simulink model "RO_Plantsimscape"  (R2020a)
settings: Solver=VariableStepAuto  StartTime=0.0  StopTime=100  RelTol=1e-3
libraries: sh_lib x108, fl_lib x76, nesl_utility x73, simulink x13
(part 1 of 4)
settings Model: Creator=cjrmx  LastModifiedBy=Kevin

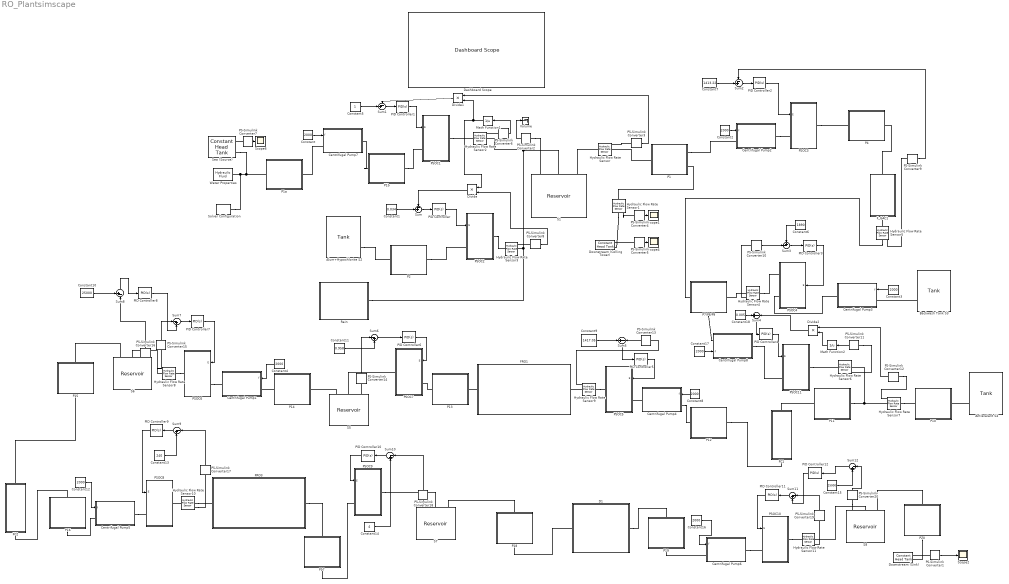
== system RO_Plantsimscape ==
  Alum+Hypochlorite S2 : sh_lib/Low-Pressure Blocks/Tank  press=1 atm  level_spec=1  tank_area=342.26 m^2  fluid_volume_tab=[0, .0028, .0065, .0114, .0176, .0252, .0344, .0436, .0512, .0574, .0623, .066, .0688, .0707, .072, .0727] m^3  fluid_level_tab=[0, .02, .04, .06, .08, .1, .12, .14, .16, .18, .2, .22, .24, .26, .28, .3] m  interp_method=1  extrap_method=1  pipe_diam=10 in  loss_coeff=1.2  g=9.81 m/s^2  min_level=1e-3 m  fluid_level_check=1  volume_specify=off  volume_priority=High  volume=20 l  volume_nominal_specify=off  volume_nominal_unit=l  volume_nominal_value=1  level_specify=on  level_priority=None  level=15 m  level_nominal_specify=off  level_nominal_unit=m  level_nominal_value=1  pipe_diam_A=0.02 m  loss_coeff_A=1.2  height_B=0.8 m  pipe_diam_B=0.02 m  loss_coeff_B=1.2  height_C=0.8 m  pipe_diam_C=0.02 m  loss_coeff_C=1.2
      settings: SourceProductBaseCode=SH  InternalSimscapePortConfiguration="{\"Bottom\":[],\"Left\":[],\"Right\":[{\"id\":\"V\",\"label\":\"V\",\"type\":\"output\"},{\"id\":\"T\",\"label\":\"T\",\"type\":\"foundation.hydraulic.hydraulic\"}],\"Top\":[]}"
  Antiscalant S4 : sh_lib/Low-Pressure Blocks/Tank  press=1 atm  level_spec=1  tank_area=20 m^2  fluid_volume_tab=[0, .0028, .0065, .0114, .0176, .0252, .0344, .0436, .0512, .0574, .0623, .066, .0688, .0707, .072, .0727] m^3  fluid_level_tab=[0, .02, .04, .06, .08, .1, .12, .14, .16, .18, .2, .22, .24, .26, .28, .3] m  interp_method=1  extrap_method=1  pipe_diam=0.02 m  loss_coeff=1.2  g=9.81 m/s^2  min_level=1e-3 m  fluid_level_check=1  volume_specify=off  volume_priority=High  volume=20 l  volume_nominal_specify=off  volume_nominal_unit=l  volume_nominal_value=1  level_specify=on  level_priority=None  level=12 m  level_nominal_specify=off  level_nominal_unit=m  level_nominal_value=1  pipe_diam_A=0.02 m  loss_coeff_A=1.2  height_B=0.8 m  pipe_diam_B=0.02 m  loss_coeff_B=1.2  height_C=0.8 m  pipe_diam_C=0.02 m  loss_coeff_C=1.2
      settings: SourceProductBaseCode=SH  InternalSimscapePortConfiguration="{\"Bottom\":[],\"Left\":[],\"Right\":[{\"id\":\"V\",\"label\":\"V\",\"type\":\"output\"},{\"id\":\"T\",\"label\":\"T\",\"type\":\"foundation.hydraulic.hydraulic\"}],\"Top\":[]}"
  Backwash Tank S3 : sh_lib/Low-Pressure Blocks/Tank  press=1 atm  level_spec=1  tank_area=12.57 m^2  fluid_volume_tab=[0, .0028, .0065, .0114, .0176, .0252, .0344, .0436, .0512, .0574, .0623, .066, .0688, .0707, .072, .0727] m^3  fluid_level_tab=[0, .02, .04, .06, .08, .1, .12, .14, .16, .18, .2, .22, .24, .26, .28, .3] m  interp_method=1  extrap_method=1  pipe_diam=0.02 m  loss_coeff=1.2  g=9.81 m/s^2  min_level=1e-3 m  fluid_level_check=1  volume_specify=off  volume_priority=High  volume=20 l  volume_nominal_specify=off  volume_nominal_unit=l  volume_nominal_value=1  level_specify=on  level_priority=None  level=8 m  level_nominal_specify=off  level_nominal_unit=m  level_nominal_value=1  pipe_diam_A=0.02 m  loss_coeff_A=1.2  height_B=0.8 m  pipe_diam_B=0.02 m  loss_coeff_B=1.2  height_C=0.8 m  pipe_diam_C=0.02 m  loss_coeff_C=1.2
      settings: SourceProductBaseCode=SH  InternalSimscapePortConfiguration="{\"Bottom\":[],\"Left\":[],\"Right\":[{\"id\":\"V\",\"label\":\"V\",\"type\":\"output\"},{\"id\":\"T\",\"label\":\"T\",\"type\":\"foundation.hydraulic.hydraulic\"}],\"Top\":[]}"
  Centrifugal Pump1 : Subsystem
      mask Display: image('$imagefile'); % Use "Edit Image" on toolstrip to change.
  Centrifugal Pump2 : Subsystem
      mask Display: image('$imagefile'); % Use "Edit Image" on toolstrip to change.
  Centrifugal Pump3 : Subsystem
      mask Display: image('$imagefile'); % Use "Edit Image" on toolstrip to change.
  Centrifugal Pump4 : Subsystem
      mask Display: image('$imagefile'); % Use "Edit Image" on toolstrip to change.
  Centrifugal Pump5 : Subsystem
      mask Display: image('$imagefile'); % Use "Edit Image" on toolstrip to change.
  Centrifugal Pump6 : Subsystem
      mask Display: image('$imagefile'); % Use "Edit Image" on toolstrip to change.
  Centrifugal Pump7 : Subsystem
      mask Display: image('$imagefile'); % Use "Edit Image" on toolstrip to change.
  Centrifugal Pump8 : Subsystem
      settings: PortSchema="{\"entries\":[{\"content\":{\"sides\":[{\"content\":{\"connectorIds\":[\"LConn1\",\"In1\"]},\"type\":\"ConnectorPlacement.EquallySpacedRectSide\",\"uuid\":\"eab26e76-19e5-4131-be01-7f1e86a3578c\"},{\"content\":{\"connectorIds\":[\"RConn1\"],\"side\":\"RIGHT\"},\"type\":\"ConnectorPlacement.EquallySpacedRectSide\",\"uuid\":\"eb3e9ef5-afdc-4988-b145-41f6f9d64aea\"},{\"content\":{\"connectorIds\":[],\"side\":\"TOP\"},\"type\":\"ConnectorPlacement.EquallySpacedRectSide\",\"uuid\":\"3eed5e1d-ef70-4ff8-841b-e6ca0040c613\"}]},\"type\":\"ConnectorPlacement.EquallySpacedConnector\",\"uuid\":\"4f5dbfc8-7a84-4fdf-87d5-9a92094a984d\"}],\"packageUris\":[\"http://schema.mathworks.com/mf0/Connector/19700101\"],\"version\":\"1.0\"}"
      mask Display: image('$imagefile'); % Use "Edit Image" on toolstrip to change.
  Constant{,2..4,8,12,16..17} (8 alike) : Constant  Value=2000
  Constant1 : Constant  Value=0.034
  Constant10 : Constant  Value=25000
  Constant11 : Constant  Value=0.958
  Constant13 : Constant  Value=240
  Constant14 : Constant  Value=4
  Constant15 : Constant  Value=25000
  Constant18 : Constant  Value=0.005
  Constant5 : Constant
  Constant6 : Constant  Value=1890
  Constant7 : Constant  Value=1413.22
  Constant9 : Constant  Value=1417.05
  D1 : Subsystem
      mask Display: image('$imagefile'); % Use "Edit Image" on toolstrip to change.
  Dashboard Scope : DashboardScope
  Divide : Product  Inputs=**
  Divide1 : Product  Inputs=**
  Divide2 : Product  Inputs=**
  Downstream (Colling Tower) : sh_lib/Low-Pressure Blocks/Constant Head Tank  press=0 Pa  fluid_level=0 m  pipe_diam=48 in  loss_coeff=1.2  g=9.81 m/s^2  volume_specify=on  volume_priority=High  volume=0 m^3  volume_nominal_specify=off  volume_nominal_unit=m^3  volume_nominal_value=1
      settings: SourceProductBaseCode=SH  InternalSimscapePortConfiguration="{\"Bottom\":[],\"Left\":[],\"Right\":[{\"id\":\"V\",\"label\":\"V\",\"type\":\"output\"},{\"id\":\"T\",\"label\":\"T\",\"type\":\"foundation.hydraulic.hydraulic\"}],\"Top\":[]}"
  Downstream (Sink) : sh_lib/Low-Pressure Blocks/Constant Head Tank  press=0 Pa  fluid_level=0 m  pipe_diam=4 in  loss_coeff=1.2  g=9.81 m/s^2  volume_specify=on  volume_priority=High  volume=0 m^3  volume_nominal_specify=off  volume_nominal_unit=m^3  volume_nominal_value=1
      settings: SourceProductBaseCode=SH  InternalSimscapePortConfiguration="{\"Bottom\":[],\"Left\":[],\"Right\":[{\"id\":\"V\",\"label\":\"V\",\"type\":\"output\"},{\"id\":\"T\",\"label\":\"T\",\"type\":\"foundation.hydraulic.hydraulic\"}],\"Top\":[]}"
  FC1 : Subsystem
      mask Display: image('$imagefile'); % Use "Edit Image" on toolstrip to change.
  FC2 : Subsystem
      mask Display: image('$imagefile'); % Use "Edit Image" on toolstrip to change.
  FRO1 : Subsystem
      mask Display: image('$imagefile'); % Use "Edit Image" on toolstrip to change.
  FRO3 : Subsystem
      mask Display: image('$imagefile'); % Use "Edit Image" on toolstrip to change.
  F_GAC1 : Subsystem
      mask Display: image('$imagefile'); % Use "Edit Image" on toolstrip to change.
  Hydraulic Flow Rate Sensor{,1..11} (12 alike) : fl_lib/Hydraulic/Hydraulic Sensors/Hydraulic Flow Rate Sensor
  Math Function1 : Math  Operator=reciprocal  SaturateOnIntegerOverflow=on
  Math Function2 : Math  Operator=reciprocal  SaturateOnIntegerOverflow=on
  P1 : Subsystem
      mask Display: image('$imagefile'); % Use "Edit Image" on toolstrip to change.
  P10 : Subsystem
      mask Display: image('$imagefile'); % Use "Edit Image" on toolstrip to change.
  P11 : Subsystem
      mask Display: image('$imagefile'); % Use "Edit Image" on toolstrip to change.
  P12 : Subsystem
      mask Display: image('$imagefile'); % Use "Edit Image" on toolstrip to change.
  P13 : Subsystem
      mask Display: image('$imagefile'); % Use "Edit Image" on toolstrip to change.
  P14 : Subsystem
      mask Display: image('$imagefile'); % Use "Edit Image" on toolstrip to change.
  P15 : Subsystem
      settings: PortSchema="{\"entries\":[{\"content\":{\"sides\":[{\"content\":{\"connectorIds\":[]},\"type\":\"ConnectorPlacement.EquallySpacedRectSide\",\"uuid\":\"46c43a71-b7fa-42e4-8d4f-3c01e3706290\"},{\"content\":{\"connectorIds\":[],\"side\":\"RIGHT\"},\"type\":\"ConnectorPlacement.EquallySpacedRectSide\",\"uuid\":\"b401084b-7303-4528-8d6f-c80864bdaeba\"},{\"content\":{\"connectorIds\":[\"LConn1\"],\"side\":\"TOP\"},\"type\":\"ConnectorPlacement.EquallySpacedRectSide\",\"uuid\":\"e7f94297-9de0-49cb-bb6c-7569d7bc8c1f\"},{\"content\":{\"connectorIds\":[\"RConn1\"],\"side\":\"BOTTOM\"},\"type\":\"ConnectorPlacement.EquallySpacedRectSide\",\"uuid\":\"17d2f97d-9159-4642-b3f0-323a39ef2445\"}]},\"type\":\"ConnectorPlacement.EquallySpacedConnector\",\"uuid\":\"a507a281-e5f3-478b-81a6-535710a561dc\"}],\"packageUris\":[\"http://schema.mathworks.com/mf0/Connector/19700101\"],\"version\":\"1.0\"}"
      mask Display: image('$imagefile'); % Use "Edit Image" on toolstrip to change.
  P16 : Subsystem
      settings: PortSchema="{\"entries\":[{\"content\":{\"sides\":[{\"content\":{\"connectorIds\":[]},\"type\":\"ConnectorPlacement.EquallySpacedRectSide\",\"uuid\":\"46c43a71-b7fa-42e4-8d4f-3c01e3706290\"},{\"content\":{\"connectorIds\":[],\"side\":\"RIGHT\"},\"type\":\"ConnectorPlacement.EquallySpacedRectSide\",\"uuid\":\"b401084b-7303-4528-8d6f-c80864bdaeba\"},{\"content\":{\"connectorIds\":[\"LConn1\"],\"side\":\"TOP\"},\"type\":\"ConnectorPlacement.EquallySpacedRectSide\",\"uuid\":\"e7f94297-9de0-49cb-bb6c-7569d7bc8c1f\"},{\"content\":{\"connectorIds\":[\"RConn1\"],\"side\":\"BOTTOM\"},\"type\":\"ConnectorPlacement.EquallySpacedRectSide\",\"uuid\":\"17d2f97d-9159-4642-b3f0-323a39ef2445\"}]},\"type\":\"ConnectorPlacement.EquallySpacedConnector\",\"uuid\":\"a507a281-e5f3-478b-81a6-535710a561dc\"}],\"packageUris\":[\"http://schema.mathworks.com/mf0/Connector/19700101\"],\"version\":\"1.0\"}"
      mask Display: image('$imagefile'); % Use "Edit Image" on toolstrip to change.
  P17 : Subsystem
      settings: PortSchema="{\"entries\":[{\"content\":{\"sides\":[{\"content\":{\"connectorIds\":[]},\"type\":\"ConnectorPlacement.EquallySpacedRectSide\",\"uuid\":\"46c43a71-b7fa-42e4-8d4f-3c01e3706290\"},{\"content\":{\"connectorIds\":[],\"side\":\"RIGHT\"},\"type\":\"ConnectorPlacement.EquallySpacedRectSide\",\"uuid\":\"b401084b-7303-4528-8d6f-c80864bdaeba\"},{\"content\":{\"connectorIds\":[\"LConn1\"],\"side\":\"TOP\"},\"type\":\"ConnectorPlacement.EquallySpacedRectSide\",\"uuid\":\"e7f94297-9de0-49cb-bb6c-7569d7bc8c1f\"},{\"content\":{\"connectorIds\":[\"RConn1\"],\"side\":\"BOTTOM\"},\"type\":\"ConnectorPlacement.EquallySpacedRectSide\",\"uuid\":\"17d2f97d-9159-4642-b3f0-323a39ef2445\"}]},\"type\":\"ConnectorPlacement.EquallySpacedConnector\",\"uuid\":\"a507a281-e5f3-478b-81a6-535710a561dc\"}],\"packageUris\":[\"http://schema.mathworks.com/mf0/Connector/19700101\"],\"version\":\"1.0\"}"
      mask Display: image('$imagefile'); % Use "Edit Image" on toolstrip to change.
  P18 : Subsystem
      settings: PortSchema="{\"entries\":[{\"content\":{\"sides\":[{\"content\":{\"connectorIds\":[]},\"type\":\"ConnectorPlacement.EquallySpacedRectSide\",\"uuid\":\"46c43a71-b7fa-42e4-8d4f-3c01e3706290\"},{\"content\":{\"connectorIds\":[],\"side\":\"RIGHT\"},\"type\":\"ConnectorPlacement.EquallySpacedRectSide\",\"uuid\":\"b401084b-7303-4528-8d6f-c80864bdaeba\"},{\"content\":{\"connectorIds\":[\"LConn1\"],\"side\":\"TOP\"},\"type\":\"ConnectorPlacement.EquallySpacedRectSide\",\"uuid\":\"e7f94297-9de0-49cb-bb6c-7569d7bc8c1f\"},{\"content\":{\"connectorIds\":[\"RConn1\"],\"side\":\"BOTTOM\"},\"type\":\"ConnectorPlacement.EquallySpacedRectSide\",\"uuid\":\"17d2f97d-9159-4642-b3f0-323a39ef2445\"}]},\"type\":\"ConnectorPlacement.EquallySpacedConnector\",\"uuid\":\"a507a281-e5f3-478b-81a6-535710a561dc\"}],\"packageUris\":[\"http://schema.mathworks.com/mf0/Connector/19700101\"],\"version\":\"1.0\"}"
      mask Display: image('$imagefile'); % Use "Edit Image" on toolstrip to change.
  P19 : Subsystem
      settings: PortSchema="{\"entries\":[{\"content\":{\"sides\":[{\"content\":{\"connectorIds\":[]},\"type\":\"ConnectorPlacement.EquallySpacedRectSide\",\"uuid\":\"46c43a71-b7fa-42e4-8d4f-3c01e3706290\"},{\"content\":{\"connectorIds\":[],\"side\":\"RIGHT\"},\"type\":\"ConnectorPlacement.EquallySpacedRectSide\",\"uuid\":\"b401084b-7303-4528-8d6f-c80864bdaeba\"},{\"content\":{\"connectorIds\":[\"LConn1\"],\"side\":\"TOP\"},\"type\":\"ConnectorPlacement.EquallySpacedRectSide\",\"uuid\":\"e7f94297-9de0-49cb-bb6c-7569d7bc8c1f\"},{\"content\":{\"connectorIds\":[\"RConn1\"],\"side\":\"BOTTOM\"},\"type\":\"ConnectorPlacement.EquallySpacedRectSide\",\"uuid\":\"17d2f97d-9159-4642-b3f0-323a39ef2445\"}]},\"type\":\"ConnectorPlacement.EquallySpacedConnector\",\"uuid\":\"a507a281-e5f3-478b-81a6-535710a561dc\"}],\"packageUris\":[\"http://schema.mathworks.com/mf0/Connector/19700101\"],\"version\":\"1.0\"}"
      mask Display: image('$imagefile'); % Use "Edit Image" on toolstrip to change.
  P1a : Subsystem
      mask Display: image('$imagefile'); % Use "Edit Image" on toolstrip to change.
  P1b : Subsystem
      mask Display: image('$imagefile'); % Use "Edit Image" on toolstrip to change.
  P2 : Subsystem
      mask Display: image('$imagefile'); % Use "Edit Image" on toolstrip to change.
  P20 : Subsystem
      settings: PortSchema="{\"entries\":[{\"content\":{\"sides\":[{\"content\":{\"connectorIds\":[]},\"type\":\"ConnectorPlacement.EquallySpacedRectSide\",\"uuid\":\"46c43a71-b7fa-42e4-8d4f-3c01e3706290\"},{\"content\":{\"connectorIds\":[],\"side\":\"RIGHT\"},\"type\":\"ConnectorPlacement.EquallySpacedRectSide\",\"uuid\":\"b401084b-7303-4528-8d6f-c80864bdaeba\"},{\"content\":{\"connectorIds\":[\"LConn1\"],\"side\":\"TOP\"},\"type\":\"ConnectorPlacement.EquallySpacedRectSide\",\"uuid\":\"e7f94297-9de0-49cb-bb6c-7569d7bc8c1f\"},{\"content\":{\"connectorIds\":[\"RConn1\"],\"side\":\"BOTTOM\"},\"type\":\"ConnectorPlacement.EquallySpacedRectSide\",\"uuid\":\"17d2f97d-9159-4642-b3f0-323a39ef2445\"}]},\"type\":\"ConnectorPlacement.EquallySpacedConnector\",\"uuid\":\"a507a281-e5f3-478b-81a6-535710a561dc\"}],\"packageUris\":[\"http://schema.mathworks.com/mf0/Connector/19700101\"],\"version\":\"1.0\"}"
      mask Display: image('$imagefile'); % Use "Edit Image" on toolstrip to change.
  P4 : Subsystem
      mask Display: image('$imagefile'); % Use "Edit Image" on toolstrip to change.
  P7/P8/P9 : Subsystem
      settings: PortSchema="{\"entries\":[{\"content\":{\"sides\":[{\"content\":{\"connectorIds\":[\"LConn1\"]},\"type\":\"ConnectorPlacement.EquallySpacedRectSide\",\"uuid\":\"c4d3b345-1774-4faf-92d9-0d4f63b9ee50\"},{\"content\":{\"connectorIds\":[\"RConn1\"],\"side\":\"RIGHT\"},\"type\":\"ConnectorPlacement.EquallySpacedRectSide\",\"uuid\":\"19590d96-e8de-4e96-ac4d-d2cb11dc0057\"},{\"content\":{\"connectorIds\":[],\"side\":\"TOP\"},\"type\":\"ConnectorPlacement.EquallySpacedRectSide\",\"uuid\":\"ab799575-47ef-4b74-8840-5dcb81dec600\"},{\"content\":{\"connectorIds\":[\"RConn2\"],\"side\":\"BOTTOM\"},\"type\":\"ConnectorPlacement.EquallySpacedRectSide\",\"uuid\":\"f791b078-7d26-4714-95a8-19c732dd4143\"}]},\"type\":\"ConnectorPlacement.EquallySpacedConnector\",\"uuid\":\"41b3ff9f-9b96-49e2-b98d-ecd42f4aada1\"}],\"packageUris\":[\"http://schema.mathworks.com/mf0/Connector/19700101\"],\"version\":\"1.0\"}"
      mask Display: image('$imagefile'); % Use "Edit Image" on toolstrip to change.
  PID Controller{,1..12} (13 alike) : simulink/Continuous/PID Controller  Controller=PID  Form=Parallel  TimeDomain=Continuous-time  UseExternalTs=off  SampleTime=-1  IntegratorMethod=Forward Euler  FilterMethod=Forward Euler  ControllerParametersSource=internal  P=1  I=1  D=0  UseFilter=on  N=100  TunerSelectOption=Transfer Function Based (PID Tuner App)  InitialConditionSource=internal  InitialConditionForIntegrator=0  InitialConditionForFilter=0  DifferentiatorICPrevScaledInput=0  ExternalReset=none  TrackingMode=off  Kt=1  LimitOutput=off  UpperSaturationLimit=inf  LowerSaturationLimit=-inf  LinearizeAsGain=on  AntiWindupMode=none  Kb=1  POutMin=[]  POutMax=[]  IOutMin=[]  IOutMax=[]  DOutMin=[]  DOutMax=[]  NOutMin=[]  NOutMax=[]  SumOutMin=[]  SumOutMax=[]  SaturationOutMin=[]  SaturationOutMax=[]  PParamMin=[]  PParamMax=[]  IParamMin=[]  IParamMax=[]  DParamMin=[]  DParamMax=[]  NParamMin=[]  NParamMax=[]  KbParamMin=[]  KbParamMax=[]  KtParamMin=[]  KtParamMax=[]  KbOutMin=[]  KbOutMax=[]  KtOutMin=[]  KtOutMax=[]  IntegratorOutMin=[]  IntegratorOutMax=[]  FilterOutMin=[]  FilterOutMax=[]  SumI1OutMin=[]  SumI1OutMax=[]  SumI2OutMin=[]  SumI2OutMax=[]  SumI3OutMin=[]  SumI3OutMax=[]  SumI4OutMin=[]  SumI4OutMax=[]  SumDOutMin=[]  SumDOutMax=[]  DifferentiatorOutMin=[]  DifferentiatorOutMax=[]  FilterDiffOutCoefMin=[]  FilterDiffOutCoefMax=[]  ReciprocalOutMin=[]  ReciprocalOutMax=[]  SumDenOutMin=[]  SumDenOutMax=[]  SumNumOutMin=[]  SumNumOutMax=[]  DivideOutMin=[]  DivideOutMax=[]  UdiffTsProdOutMin=[]  UdiffTsProdOutMax=[]  NTsProdOutMin=[]  NTsProdOutMax=[]  UintegralTsProdOutMin=[]  UintegralTsProdOutMax=[]  UngainTsProdOutMin=[]  UngainTsProdOutMax=[]  IntegratorContinuousStateAttributes=''  IntegratorStateMustResolveToSignalObject=off  IntegratorRTWStateStorageClass=Auto  FilterContinuousStateAttributes=''  FilterStateMustResolveToSignalObject=off  FilterRTWStateStorageClass=Auto  ParallelPVariant=InternalParameters  IdealPVariant=Disabled  IVariant=InternalParameters  DVariant=InternalParameters  IntegratorVariant=Continuous  SatVariant=Disabled  AWVariant=Passthrough  PCopyVariant=Disabled  TRVariant=Disabled  FdbkBlocksVariant=Forward  IdealPFdbkVariant=Disabled  SatFdbkVariant=Disabled  DerivativeFilterVariant=ContFilter  NVariant=InternalParameters  NCopyVariant=Disabled  FilterICVariant=InternalICsFilter  IntegratorICVariant=InternalICs  ExternalResetVariant=Disabled  TRSumVariant=Passthrough  SumFdbkVariant=Disabled  SumVariant=Sum_PID  TsampFilterVariant=InternalTs  TsampNgainVariant=Passthrough  TsampIntegralVariant=Passthrough
  PS-Simulink Converter{1..20} (20 alike) : nesl_utility/PS-Simulink Converter  PhysicalDomain=network_engine_domain  SubClassName=ps_output  LeftPortType=input  RightPortType=output  PseudoPeriodic=off  Frequencies=[]  Unit=1  AffineConversion=off
  PSOC1 : Subsystem
      mask Display: image('$imagefile'); % Use "Edit Image" on toolstrip to change.
  PSOC10 : Subsystem
      mask Display: image('$imagefile'); % Use "Edit Image" on toolstrip to change.
  PSOC11 : Subsystem
      mask Display: image('$imagefile'); % Use "Edit Image" on toolstrip to change.
  PSOC2 : Subsystem
      mask Display: image('$imagefile'); % Use "Edit Image" on toolstrip to change.
  PSOC3 : Subsystem
      mask Display: image('$imagefile'); % Use "Edit Image" on toolstrip to change.
  PSOC4 : Subsystem
      mask Display: image('$imagefile'); % Use "Edit Image" on toolstrip to change.
  PSOC5 : Subsystem
      mask Display: image('$imagefile'); % Use "Edit Image" on toolstrip to change.
  PSOC6 : Subsystem
      mask Display: image('$imagefile'); % Use "Edit Image" on toolstrip to change.
  PSOC7 : Subsystem
      mask Display: image('$imagefile'); % Use "Edit Image" on toolstrip to change.
  PSOC8 : Subsystem
      mask Display: image('$imagefile'); % Use "Edit Image" on toolstrip to change.
  PSOC9 : Subsystem
      mask Display: image('$imagefile'); % Use "Edit Image" on toolstrip to change.
  Rain : Subsystem
      mask Display: image('$imagefile'); % Use "Edit Image" on toolstrip to change.
  S1 : sh_lib/Hydraulic Utilities/Reservoir  press=1 atm  init_volume=20000 m^3  ret_diam=48 in  loss_coeff=1
      settings: SourceProductBaseCode=SH  InternalSimscapePortConfiguration="{\"Bottom\":[],\"Left\":[{\"id\":\"V\",\"label\":\"V\",\"type\":\"output\"},{\"id\":\"P\",\"label\":\"P\",\"type\":\"foundation.hydraulic.hydraulic\"},{\"id\":\"R\",\"label\":\"R\",\"type\":\"foundation.hydraulic.hydraulic\"}],\"Right\":[],\"Top\":[]}"
  S5 : sh_lib/Hydraulic Utilities/Reservoir  press=1 atm  init_volume=1 m^3  ret_diam=4 in  loss_coeff=1
      settings: SourceProductBaseCode=SH  InternalSimscapePortConfiguration="{\"Bottom\":[],\"Left\":[{\"id\":\"V\",\"label\":\"V\",\"type\":\"output\"},{\"id\":\"P\",\"label\":\"P\",\"type\":\"foundation.hydraulic.hydraulic\"},{\"id\":\"R\",\"label\":\"R\",\"type\":\"foundation.hydraulic.hydraulic\"}],\"Right\":[],\"Top\":[]}"
  S6 : sh_lib/Hydraulic Utilities/Reservoir  press=1 atm  init_volume=27000 m^3  ret_diam=4 in  loss_coeff=1
      settings: SourceProductBaseCode=SH  InternalSimscapePortConfiguration="{\"Bottom\":[],\"Left\":[{\"id\":\"V\",\"label\":\"V\",\"type\":\"output\"},{\"id\":\"P\",\"label\":\"P\",\"type\":\"foundation.hydraulic.hydraulic\"},{\"id\":\"R\",\"label\":\"R\",\"type\":\"foundation.hydraulic.hydraulic\"}],\"Right\":[],\"Top\":[]}"
  S7 : sh_lib/Hydraulic Utilities/Reservoir  press=1 atm  init_volume=4 m^3  ret_diam=4 in  loss_coeff=1
      settings: SourceProductBaseCode=SH  InternalSimscapePortConfiguration="{\"Bottom\":[],\"Left\":[{\"id\":\"V\",\"label\":\"V\",\"type\":\"output\"},{\"id\":\"P\",\"label\":\"P\",\"type\":\"foundation.hydraulic.hydraulic\"},{\"id\":\"R\",\"label\":\"R\",\"type\":\"foundation.hydraulic.hydraulic\"}],\"Right\":[],\"Top\":[]}"
  S8 : sh_lib/Hydraulic Utilities/Reservoir  press=1 atm  init_volume=27000 m^3  ret_diam=4 in  loss_coeff=1
      settings: SourceProductBaseCode=SH  InternalSimscapePortConfiguration="{\"Bottom\":[],\"Left\":[{\"id\":\"V\",\"label\":\"V\",\"type\":\"output\"},{\"id\":\"P\",\"label\":\"P\",\"type\":\"foundation.hydraulic.hydraulic\"},{\"id\":\"R\",\"label\":\"R\",\"type\":\"foundation.hydraulic.hydraulic\"}],\"Right\":[],\"Top\":[]}"
  Scope{1..2,4,6} (4 alike) : Scope
  Sea (Source) : sh_lib/Low-Pressure Blocks/Constant Head Tank  press=1 atm  fluid_level=5000 m  pipe_diam=48 in  loss_coeff=1.2  g=9.81 m/s^2  volume_specify=on  volume_priority=High  volume=10000 m^3  volume_nominal_specify=off  volume_nominal_unit=m^3  volume_nominal_value=1
      settings: SourceProductBaseCode=SH  InternalSimscapePortConfiguration="{\"Bottom\":[],\"Left\":[],\"Right\":[{\"id\":\"V\",\"label\":\"V\",\"type\":\"output\"},{\"id\":\"T\",\"label\":\"T\",\"type\":\"foundation.hydraulic.hydraulic\"}],\"Top\":[]}"
  Solver Configuration : nesl_utility/Solver Configuration  PhysicalDomain=network_engine_domain  SubClassName=solver  LeftPortType=input  RightPortType=generic  Tones=[]  Harmonics=[]  SimulateNoise=off  Profile=off  UseLocalSampling=off  EnableSwitchedLinearOptims=on  FrequencyDomain=off  UseCCode=off  RelTol=0.001  AbsTol=1e-06  MinStep=1e-09  ToWorkspace=off  RevertToSquareIcSolve=off  NumHomotopyIterations=100  PhasorMode=off  PhasorModeNumHarmonics=1  DoDC=off  ResidualTolerance=1e-9  UseLocalSolver=off  LocalSolverChoice=NE_BACKWARD_EULER_ADVANCER  LocalSolverSampleTime=.001  DoFixedCost=off  MaxNonlinIter=3  MaxModeIter=2  LinearAlgebra=auto  EquationFormulation=NE_TIME_EF  DelaysMemoryBudget=1024  AutomaticFiltering=on  FilteringTimeConstant=0.001  PartitionStorageMethod=AS_NEEDED  PartitionMemoryBudget=1024  PartitionMethod=FAST
  Sum : Sum  Inputs=-+|
  Sum1 : Sum  Inputs=-+|
  Sum{6..7,9..12} (6 alike) : Sum  Inputs=|-+
  Sum2 : Sum  Inputs=-+|
  Sum3 : Sum  Inputs=+-|
  Sum4 : Sum  Inputs=+|-
  Sum5 : Sum  Inputs=+|-
  Sum8 : Sum  Inputs=+-|
  Volume : Terminator
  Water Properties : sh_lib/Hydraulic Utilities/Hydraulic Fluid  DataSource=1  SelFluid=24  SysTemp=1  TrapAir=0.001  ViscDerFactor=1  range_error=2
  wires:
  Constant/1 -> Centrifugal Pump7/1(f)
  PS-Simulink Converter1/1 -> Scope2/1
  PS-Simulink Converter3/1 -> Divide1/1
  PS-Simulink Converter2/1 -> Volume/1
  PS-Simulink Converter4/1 -> Scope1/1
  PS-Simulink Converter5/1 -> Scope4/1
  Constant3/1 -> Centrifugal Pump3/1(f)
  Constant8/1 -> Centrifugal Pump4/1(f)
  Constant4/1 -> Centrifugal Pump1/1(f)
  Constant12/1 -> Centrifugal Pump5/1(f)
  Constant16/1 -> Centrifugal Pump6/1(f)
  PS-Simulink Converter7/1 -> Scope6/1
  PS-Simulink Converter6/1 -> Math Function1/1
  Constant2/1 -> Centrifugal Pump2/1(f)
  Constant1/1 -> Sum/2
  Sum/1 -> PID Controller/1
  PID Controller/1 -> PSOC2/1(E)
  Divide/1 -> Sum/1
  PS-Simulink Converter8/1 -> Divide/2
  Math Function1/1 -> Divide1/2, Divide/1
  Sum1/1 -> PID Controller1/1
  Constant5/1 -> Sum1/2
  PID Controller1/1 -> PSOC1/1(E)
  Divide1/1 -> Sum1/1
  Constant7/1 -> Sum2/2
  Sum2/1 -> PID Controller2/1
  PID Controller2/1 -> PSOC3/1(E)
  PS-Simulink Converter9/1 -> Sum2/1
  PS-Simulink Converter10/1 -> Sum3/2
  Constant6/1 -> Sum3/1
  Sum3/1 -> PID Controller3/1
  PID Controller3/1 -> PSOC4/1(E)
  Constant17/1 -> Centrifugal Pump8/1(f)
  PID Controller4/1 -> PSOC11/1(E)
  Sum4/1 -> PID Controller4/1
  Constant18/1 -> Sum4/1
  PS-Simulink Converter11/1 -> Math Function2/1
  Divide2/1 -> Sum4/2
  Math Function2/1 -> Divide2/2
  PS-Simulink Converter12/1 -> Divide2/1
  PID Controller5/1 -> PSOC5/1(E)
  Sum5/1 -> PID Controller5/1
  Constant9/1 -> Sum5/1
  PS-Simulink Converter13/1 -> Sum5/2
  PID Controller6/1 -> PSOC7/1(E)
  Sum6/1 -> PID Controller6/1
  PS-Simulink Converter14/1 -> Sum6/1
  Constant11/1 -> Sum6/2
  PID Controller7/1 -> PSOC6/1(E)
  PS-Simulink Converter15/1 -> Sum7/1
  Sum7/1 -> PID Controller7/1
  PID Controller8/1 -> Sum7/2
  Sum8/1 -> PID Controller8/1
  PS-Simulink Converter16/1 -> Sum8/2
  Constant10/1 -> Sum8/1
  PS-Simulink Converter17/1 -> Sum9/1
  Sum9/1 -> PID Controller9/1
  PID Controller9/1 -> PSOC8/1(E)
  Constant13/1 -> Sum9/2
  PS-Simulink Converter18/1 -> Sum10/1
  Sum10/1 -> PID Controller10/1
  PID Controller10/1 -> PSOC9/1(E)
  Constant14/1 -> Sum10/2
  Sum11/1 -> PID Controller11/1
  PS-Simulink Converter19/1 -> Sum11/1
  PID Controller11/1 -> PSOC10/1(E)
  PS-Simulink Converter20/1 -> Sum12/1
  Sum12/1 -> PID Controller12/1
  PID Controller12/1 -> Sum11/2
  Constant15/1 -> Sum12/2
  connections:
  PS-Simulink Converter2/LConn1 -- S1/LConn1
  PS-Simulink Converter1/LConn1 -- Downstream (Sink)/RConn1
  PS-Simulink Converter3/LConn1 -- Hydraulic Flow Rate Sensor/RConn1
  Sea (Source)/RConn2 -- P1a/LConn1 -- Solver Configuration/RConn1 -- Water Properties/RConn1
  P11/LConn1 -- Hydraulic Flow Rate Sensor7/RConn2 -- Hydraulic Flow Rate Sensor6/RConn2
  Alum+Hypochlorite S2/RConn2 -- P2/LConn1
  P2/RConn1 -- PSOC2/LConn1
  Hydraulic Flow Rate Sensor1/RConn1 -- PS-Simulink Converter4/LConn1
  Hydraulic Flow Rate Sensor1/RConn2 -- Downstream (Colling Tower)/RConn2
  PS-Simulink Converter5/LConn1 -- Downstream (Colling Tower)/RConn1
  PSOC3/RConn1 -- P4/LConn1
  Centrifugal Pump3/RConn1 -- PSOC4/RConn2
  Backwash Tank S3/RConn2 -- Centrifugal Pump3/LConn1
  Antiscalant S4/RConn2 -- P10/LConn1
  P11/RConn1 -- FC1/LConn1
  P12/LConn1 -- FC1/RConn1
  S5/LConn3 -- P14/LConn1
  Centrifugal Pump4/LConn1 -- P12/RConn1
  Centrifugal Pump4/RConn1 -- PSOC5/LConn1
  PSOC6/LConn1 -- Centrifugal Pump1/RConn1
  P14/RConn1 -- Centrifugal Pump1/LConn1
  P13/RConn1 -- PSOC7/LConn1
  PSOC7/RConn1 -- S5/LConn2
  S6/LConn3 -- P15/LConn1
  FC2/LConn1 -- P15/RConn1
  Centrifugal Pump5/RConn1 -- PSOC8/LConn1
  PSOC9/RConn1 -- S7/LConn2
  Centrifugal Pump6/RConn1 -- PSOC10/LConn1
  P16/LConn1 -- FC2/RConn1
  P16/RConn1 -- Centrifugal Pump5/LConn1
  FRO3/RConn1 -- P17/LConn1
  P17/RConn1 -- PSOC9/LConn1
  S7/LConn3 -- P18/LConn1
  P18/RConn1 -- D1/LConn1
  P19/RConn1 -- Centrifugal Pump6/LConn1
  P20/RConn1 -- Downstream (Sink)/RConn2
  Hydraulic Flow Rate Sensor3/RConn2 -- Rain/RConn1 -- S1/LConn2 -- Hydraulic Flow Rate Sensor2/RConn2
  Hydraulic Flow Rate Sensor/LConn1 -- S1/LConn3
  PS-Simulink Converter7/LConn1 -- Sea (Source)/RConn1
  PSOC1/RConn1 -- Hydraulic Flow Rate Sensor2/LConn1
  Centrifugal Pump7/LConn1 -- P1a/RConn1
  P1b/LConn1 -- Centrifugal Pump7/RConn1
  P1b/RConn1 -- PSOC1/LConn1
  PSOC2/RConn1 -- Hydraulic Flow Rate Sensor3/LConn1
  PS-Simulink Converter6/LConn1 -- Hydraulic Flow Rate Sensor2/RConn1
  PS-Simulink Converter8/LConn1 -- Hydraulic Flow Rate Sensor3/RConn1
  Centrifugal Pump2/RConn1 -- PSOC3/LConn1
  P1/RConn1 -- Centrifugal Pump2/LConn1
  P1/LConn1 -- Hydraulic Flow Rate Sensor/RConn2
  Hydraulic Flow Rate Sensor1/LConn1 -- P1/RConn2
  F_GAC1/LConn1 -- P4/RConn1
  PS-Simulink Converter9/LConn1 -- Hydraulic Flow Rate Sensor5/RConn1
  Hydraulic Flow Rate Sensor5/LConn1 -- F_GAC1/RConn1
  Hydraulic Flow Rate Sensor5/RConn2 -- P7/P8/P9/LConn1
  Hydraulic Flow Rate Sensor4/LConn1 -- PSOC4/RConn1
  Hydraulic Flow Rate Sensor4/RConn2 -- P7/P8/P9/RConn1
  Hydraulic Flow Rate Sensor4/RConn1 -- PS-Simulink Converter10/LConn1
  P7/P8/P9/RConn2 -- Centrifugal Pump8/LConn1
  Centrifugal Pump8/RConn1 -- PSOC11/LConn1
  PSOC11/RConn1 -- Hydraulic Flow Rate Sensor6/LConn1
  PS-Simulink Converter11/LConn1 -- Hydraulic Flow Rate Sensor6/RConn1
  Hydraulic Flow Rate Sensor7/LConn1 -- P10/RConn1
  PS-Simulink Converter12/LConn1 -- Hydraulic Flow Rate Sensor7/RConn1
  FRO1/RConn1 -- P13/LConn1
  Hydraulic Flow Rate Sensor9/RConn2 -- FRO1/LConn1
  Hydraulic Flow Rate Sensor9/LConn1 -- PSOC5/RConn1
  Hydraulic Flow Rate Sensor9/RConn1 -- PS-Simulink Converter13/LConn1
  S5/LConn1 -- PS-Simulink Converter14/LConn1
  Hydraulic Flow Rate Sensor8/LConn1 -- PSOC6/RConn1
  Hydraulic Flow Rate Sensor8/RConn2 -- S6/LConn2
  Hydraulic Flow Rate Sensor8/RConn1 -- PS-Simulink Converter15/LConn1
  Hydraulic Flow Rate Sensor10/LConn1 -- PSOC8/RConn1
  Hydraulic Flow Rate Sensor10/RConn2 -- FRO3/LConn1
  Hydraulic Flow Rate Sensor10/RConn1 -- PS-Simulink Converter17/LConn1
  PS-Simulink Converter18/LConn1 -- S7/LConn1
  PSOC10/RConn1 -- Hydraulic Flow Rate Sensor11/LConn1
  D1/RConn1 -- P19/LConn1
  Hydraulic Flow Rate Sensor11/RConn2 -- S8/LConn2
  S8/LConn3 -- P20/LConn1
  Hydraulic Flow Rate Sensor11/RConn1 -- PS-Simulink Converter19/LConn1
  PS-Simulink Converter20/LConn1 -- S8/LConn1

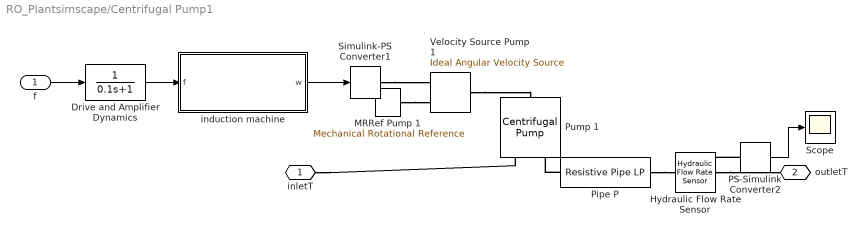
== system RO_Plantsimscape/Centrifugal Pump1 ==
  f : Inport
  Drive and Amplifier Dynamics : TransferFcn  Denominator=[0.1 1]
  Hydraulic Flow Rate Sensor : fl_lib/Hydraulic/Hydraulic Sensors/Hydraulic Flow Rate Sensor
  MRRef Pump 1 : fl_lib/Mechanical/Rotational Elements/Mechanical Rotational Reference
  PS-Simulink Converter2 : nesl_utility/PS-Simulink Converter  PhysicalDomain=network_engine_domain  SubClassName=ps_output  LeftPortType=input  RightPortType=output  PseudoPeriodic=off  Frequencies=[]  Unit=1  AffineConversion=off
  Pipe P : sh_lib/Low-Pressure Blocks/Resistive Pipe LP  cs_type=1  d_in=112.1660 mm  area=1e-04 m^2  D_h=0.0112 m  s_factor=64  length=8.1 m  length_ad=1 m  roughness=0.005 mm  Re_lam=2e+03  Re_turb=4e+03  elevation_A=45 m  elevation_B=45 m  g=9.80665 m/s^2  pressure_drop_specify=off  pressure_drop_priority=None  pressure_drop=0 Pa  pressure_drop_nominal_specify=off  pressure_drop_nominal_unit=Pa  pressure_drop_nominal_value=1  flow_rate_specify=off  flow_rate_priority=None  flow_rate=0 m^3/s  flow_rate_nominal_specify=off  flow_rate_nominal_unit=m^3/s  flow_rate_nominal_value=1
      settings: SourceProductBaseCode=SH  InternalSimscapePortConfiguration="{\"Bottom\":[],\"Left\":[{\"id\":\"A\",\"label\":\"A\",\"type\":\"foundation.hydraulic.hydraulic\"}],\"Right\":[{\"id\":\"B\",\"label\":\"B\",\"type\":\"foundation.hydraulic.hydraulic\"}],\"Top\":[]}"
  Pump 1 : sh_lib/Pumps and Motors/Centrifugal Pump  mdl_type=2  c_1=326.8 Pa/(kg/m^3)  c_2=3.104e+04 Pa*s/kg  c_3=1.097e+07 Pa*s^2/(kg*m^3)  c_4=2.136e+05 Pa*s^2/(kg*m^3)  c_f=0.8  design_del=130 lpm  ref_velocity=1.77e+03 rpm  ref_density=1000 kg/m^3  leak_resistance=1e+8 Pa/(m^3/s)  T_const=0.1 N*m  trq_press_coeff=1e-6 N*m/Pa  pump_del_1D="[0    0.0032    0.0063    0.0095    0.0126    0.0158] m^3/s"  press_diff_1D="[4.4851    4.3655    4.1413    3.7376    2.9901    1.7940] bar"  pump_del_power_1D="[0    0.0032    0.0063    0.0095    0.0126    0.0158] m^3/s"  power_1D="[0\t2116.60000000000\t3727.20000000000\t4734.30000000000\t5232.70000000000\t4360.90000000000] W"  pump_vel_2D="[  3.2e+03 3.3e+03 3.4e+03 3.5e+03 ] rpm"  pump_del_2D="[  0 50 100 150 200 250 300 350 ] lpm"  press_diff_2D="[  8.3 8.8 9.3 9.9 ; 7.8 8.3 8.8 9.4 ; 7.2 7.6 8.2 8.7 ; 6.5 7 7.5 8 ; 5.6 6.1 6.6 7.1 ; 4.7 5.2 5.7 6.2 ; 3.4 4 4.4 4.9 ; 2.3 2.7 3.4 3.6 ; ] bar"  pump_del_power_2D="[  0 50 100 150 200 250 300 350 ] lpm"  power_2D="[  1.223e+03 1.341e+03 1.467e+03 1.6e+03 ; 1.414e+03 1.551e+03 1.696e+03 1.85e+03 ; 1.636e+03 1.794e+03 1.962e+03 2.14e+03 ; 1.941e+03 2.129e+03 2.326e+03 2.54e+03 ; 2.224e+03 2.439e+03 2.66e+03 2.91e+03 ; 2.453e+03 2.691e+03 2.947e+03 3.21e+03 ; 2.757e+03 3.024e+03 3.307e+03 3.608e+03 ; 2.945e+03 3.23e+03 3.533e+03 3.854e+03 ; ] W"  omega_threshold=1e-9 rad/s  interp_method=2  extrap_method=1
      settings: SourceProductBaseCode=SH  InternalSimscapePortConfiguration="{\"Bottom\":[],\"Left\":[{\"id\":\"S\",\"label\":\"S\",\"type\":\"foundation.mechanical.rotational.rotational\"}],\"Right\":[{\"id\":\"P\",\"label\":\"P\",\"type\":\"foundation.hydraulic.hydraulic\"},{\"id\":\"T\",\"label\":\"T\",\"type\":\"foundation.hydraulic.hydraulic\"}],\"Top\":[]}"
  Scope : Scope
  Simulink-PS Converter1 : nesl_utility/Simulink-PS Converter  PhysicalDomain=network_engine_domain  SubClassName=ps_input  LeftPortType=input  RightPortType=output  PseudoPeriodic=off  Frequencies=[]  NoiseDistribution=none  NoiseParameters=[]  Unit=rpm  AffineConversion=off  FilteringAndDerivatives=zero  SimscapeFilterOrder=1  InputFilterTimeConstant=.001  UdotUserProvided=0
  Velocity Source Pump 1 : fl_lib/Mechanical/Mechanical Sources/Ideal Angular Velocity Source
  induction machine : Subsystem
  inletT : PMIOPort  Side=Left
  outletT : PMIOPort  Port=2  Side=Right
  wires:
  f/1 -> Drive and Amplifier Dynamics/1
  induction machine/1(w) -> Simulink-PS Converter1/1
  Drive and Amplifier Dynamics/1 -> induction machine/1(f)
  PS-Simulink Converter2/1 -> Scope/1
  connections:
  Velocity Source Pump 1/LConn1 -- Pump 1/LConn1
  MRRef Pump 1/LConn1 -- Velocity Source Pump 1/RConn2
  inletT/RConn1 -- Pump 1/RConn2
  Pipe P/LConn1 -- Pump 1/RConn1
  Simulink-PS Converter1/RConn1 -- Velocity Source Pump 1/RConn1
  Pipe P/RConn1 -- Hydraulic Flow Rate Sensor/LConn1
  Hydraulic Flow Rate Sensor/RConn2 -- outletT/RConn1
  PS-Simulink Converter2/LConn1 -- Hydraulic Flow Rate Sensor/RConn1

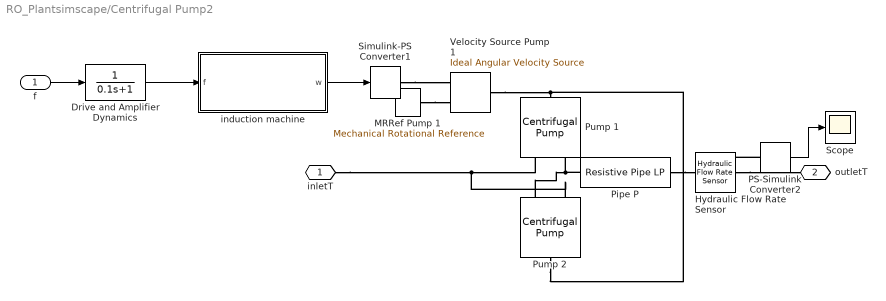
== system RO_Plantsimscape/Centrifugal Pump2 ==
  f : Inport
  Drive and Amplifier Dynamics : TransferFcn  Denominator=[0.1 1]
  Hydraulic Flow Rate Sensor : fl_lib/Hydraulic/Hydraulic Sensors/Hydraulic Flow Rate Sensor
  MRRef Pump 1 : fl_lib/Mechanical/Rotational Elements/Mechanical Rotational Reference
  PS-Simulink Converter2 : nesl_utility/PS-Simulink Converter  PhysicalDomain=network_engine_domain  SubClassName=ps_output  LeftPortType=input  RightPortType=output  PseudoPeriodic=off  Frequencies=[]  Unit=1  AffineConversion=off
  Pipe P : sh_lib/Low-Pressure Blocks/Resistive Pipe LP  cs_type=1  d_in=48 in  area=1e-04 m^2  D_h=0.0112 m  s_factor=7.15e-02  length=8.1 m  length_ad=1 m  roughness=0.005 mm  Re_lam=2e+03  Re_turb=4e+03  elevation_A=45 m  elevation_B=45 m  g=9.80665 m/s^2  pressure_drop_specify=off  pressure_drop_priority=None  pressure_drop=0 Pa  pressure_drop_nominal_specify=off  pressure_drop_nominal_unit=Pa  pressure_drop_nominal_value=1  flow_rate_specify=off  flow_rate_priority=None  flow_rate=0 m^3/s  flow_rate_nominal_specify=off  flow_rate_nominal_unit=m^3/s  flow_rate_nominal_value=1
      settings: SourceProductBaseCode=SH  InternalSimscapePortConfiguration="{\"Bottom\":[],\"Left\":[{\"id\":\"A\",\"label\":\"A\",\"type\":\"foundation.hydraulic.hydraulic\"}],\"Right\":[{\"id\":\"B\",\"label\":\"B\",\"type\":\"foundation.hydraulic.hydraulic\"}],\"Top\":[]}"
  Pump 1 : sh_lib/Pumps and Motors/Centrifugal Pump  mdl_type=1  c_1=3.268e+15 Pa/(kg/m^3)  c_2=3.104e+08 Pa*s/kg  c_3=1.097e+011 Pa*s^2/(kg*m^3)  c_4=2.136e+09 Pa*s^2/(kg*m^3)  c_f=0.8  design_del=1000 gpm  ref_velocity=1.77e+03 rpm  ref_density=1000 kg/m^3  leak_resistance=1e+8 Pa/(m^3/s)  T_const=1000 N*m  trq_press_coeff=1e-6 N*m/Pa  pump_del_1D="[0    0.0032    0.0063    0.0095    0.0126    0.0158] m^3/s"  press_diff_1D="[4.4851    4.3655    4.1413    3.7376    2.9901    1.7940] bar"  pump_del_power_1D="[0    0.0032    0.0063    0.0095    0.0126    0.0158] m^3/s"  power_1D="[0\t2116.60000000000\t3727.20000000000\t4734.30000000000\t5232.70000000000\t4360.90000000000] W"  pump_vel_2D="[  3.2e+03 3.3e+03 3.4e+03 3.5e+03 ] rpm"  pump_del_2D="[  0 50 100 150 200 250 300 350 ] lpm"  press_diff_2D="[  8.3 8.8 9.3 9.9 ; 7.8 8.3 8.8 9.4 ; 7.2 7.6 8.2 8.7 ; 6.5 7 7.5 8 ; 5.6 6.1 6.6 7.1 ; 4.7 5.2 5.7 6.2 ; 3.4 4 4.4 4.9 ; 2.3 2.7 3.4 3.6 ; ] bar"  pump_del_power_2D="[  0 50 100 150 200 250 300 350 ] lpm"  power_2D="[  1.223e+03 1.341e+03 1.467e+03 1.6e+03 ; 1.414e+03 1.551e+03 1.696e+03 1.85e+03 ; 1.636e+03 1.794e+03 1.962e+03 2.14e+03 ; 1.941e+03 2.129e+03 2.326e+03 2.54e+03 ; 2.224e+03 2.439e+03 2.66e+03 2.91e+03 ; 2.453e+03 2.691e+03 2.947e+03 3.21e+03 ; 2.757e+03 3.024e+03 3.307e+03 3.608e+03 ; 2.945e+03 3.23e+03 3.533e+03 3.854e+03 ; ] W"  omega_threshold=1e-9 rad/s  interp_method=2  extrap_method=1
      settings: SourceProductBaseCode=SH  InternalSimscapePortConfiguration="{\"Bottom\":[],\"Left\":[{\"id\":\"S\",\"label\":\"S\",\"type\":\"foundation.mechanical.rotational.rotational\"}],\"Right\":[{\"id\":\"P\",\"label\":\"P\",\"type\":\"foundation.hydraulic.hydraulic\"},{\"id\":\"T\",\"label\":\"T\",\"type\":\"foundation.hydraulic.hydraulic\"}],\"Top\":[]}"
  Pump 2 : sh_lib/Pumps and Motors/Centrifugal Pump  mdl_type=1  c_1=3.268e+15 Pa/(kg/m^3)  c_2=3.104e+08 Pa*s/kg  c_3=1.097e+011 Pa*s^2/(kg*m^3)  c_4=2.136e+09 Pa*s^2/(kg*m^3)  c_f=0.8  design_del=1000 gpm  ref_velocity=1.77e+03 rpm  ref_density=1000 kg/m^3  leak_resistance=1e+8 Pa/(m^3/s)  T_const=1000 N*m  trq_press_coeff=1e-6 N*m/Pa  pump_del_1D="[0    0.0032    0.0063    0.0095    0.0126    0.0158] m^3/s"  press_diff_1D="[4.4851    4.3655    4.1413    3.7376    2.9901    1.7940] bar"  pump_del_power_1D="[0    0.0032    0.0063    0.0095    0.0126    0.0158] m^3/s"  power_1D="[0\t2116.60000000000\t3727.20000000000\t4734.30000000000\t5232.70000000000\t4360.90000000000] W"  pump_vel_2D="[  3.2e+03 3.3e+03 3.4e+03 3.5e+03 ] rpm"  pump_del_2D="[  0 50 100 150 200 250 300 350 ] lpm"  press_diff_2D="[  8.3 8.8 9.3 9.9 ; 7.8 8.3 8.8 9.4 ; 7.2 7.6 8.2 8.7 ; 6.5 7 7.5 8 ; 5.6 6.1 6.6 7.1 ; 4.7 5.2 5.7 6.2 ; 3.4 4 4.4 4.9 ; 2.3 2.7 3.4 3.6 ; ] bar"  pump_del_power_2D="[  0 50 100 150 200 250 300 350 ] lpm"  power_2D="[  1.223e+03 1.341e+03 1.467e+03 1.6e+03 ; 1.414e+03 1.551e+03 1.696e+03 1.85e+03 ; 1.636e+03 1.794e+03 1.962e+03 2.14e+03 ; 1.941e+03 2.129e+03 2.326e+03 2.54e+03 ; 2.224e+03 2.439e+03 2.66e+03 2.91e+03 ; 2.453e+03 2.691e+03 2.947e+03 3.21e+03 ; 2.757e+03 3.024e+03 3.307e+03 3.608e+03 ; 2.945e+03 3.23e+03 3.533e+03 3.854e+03 ; ] W"  omega_threshold=1e-9 rad/s  interp_method=2  extrap_method=1
      settings: SourceProductBaseCode=SH  InternalSimscapePortConfiguration="{\"Bottom\":[],\"Left\":[{\"id\":\"S\",\"label\":\"S\",\"type\":\"foundation.mechanical.rotational.rotational\"}],\"Right\":[{\"id\":\"P\",\"label\":\"P\",\"type\":\"foundation.hydraulic.hydraulic\"},{\"id\":\"T\",\"label\":\"T\",\"type\":\"foundation.hydraulic.hydraulic\"}],\"Top\":[]}"
  Scope : Scope
  Simulink-PS Converter1 : nesl_utility/Simulink-PS Converter  PhysicalDomain=network_engine_domain  SubClassName=ps_input  LeftPortType=input  RightPortType=output  PseudoPeriodic=off  Frequencies=[]  NoiseDistribution=none  NoiseParameters=[]  Unit=rpm  AffineConversion=off  FilteringAndDerivatives=zero  SimscapeFilterOrder=1  InputFilterTimeConstant=.001  UdotUserProvided=0
  Velocity Source Pump 1 : fl_lib/Mechanical/Mechanical Sources/Ideal Angular Velocity Source
  induction machine : Subsystem
  inletT : PMIOPort  Side=Left
  outletT : PMIOPort  Port=2  Side=Right
  wires:
  f/1 -> Drive and Amplifier Dynamics/1
  induction machine/1(w) -> Simulink-PS Converter1/1
  Drive and Amplifier Dynamics/1 -> induction machine/1(f)
  PS-Simulink Converter2/1 -> Scope/1
  connections:
  Velocity Source Pump 1/LConn1 -- Pump 2/LConn1 -- Pump 1/LConn1
  MRRef Pump 1/LConn1 -- Velocity Source Pump 1/RConn2
  inletT/RConn1 -- Pump 2/RConn2 -- Pump 1/RConn2
  Pipe P/LConn1 -- Pump 1/RConn1 -- Pump 2/RConn1
  Simulink-PS Converter1/RConn1 -- Velocity Source Pump 1/RConn1
  Pipe P/RConn1 -- Hydraulic Flow Rate Sensor/LConn1
  Hydraulic Flow Rate Sensor/RConn2 -- outletT/RConn1
  PS-Simulink Converter2/LConn1 -- Hydraulic Flow Rate Sensor/RConn1

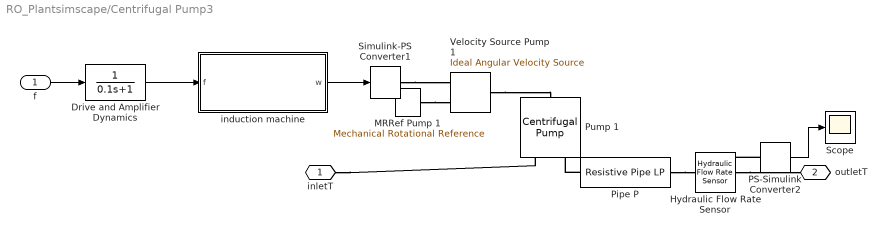
== system RO_Plantsimscape/Centrifugal Pump3 ==
  f : Inport
  Drive and Amplifier Dynamics : TransferFcn  Denominator=[0.1 1]
  Hydraulic Flow Rate Sensor : fl_lib/Hydraulic/Hydraulic Sensors/Hydraulic Flow Rate Sensor
  MRRef Pump 1 : fl_lib/Mechanical/Rotational Elements/Mechanical Rotational Reference
  PS-Simulink Converter2 : nesl_utility/PS-Simulink Converter  PhysicalDomain=network_engine_domain  SubClassName=ps_output  LeftPortType=input  RightPortType=output  PseudoPeriodic=off  Frequencies=[]  Unit=1  AffineConversion=off
  Pipe P : sh_lib/Low-Pressure Blocks/Resistive Pipe LP  cs_type=1  d_in=112.1660 mm  area=1e-04 m^2  D_h=0.0112 m  s_factor=64  length=8.1 m  length_ad=1 m  roughness=0.005 mm  Re_lam=2e+03  Re_turb=4e+03  elevation_A=45 m  elevation_B=45 m  g=9.80665 m/s^2  pressure_drop_specify=off  pressure_drop_priority=None  pressure_drop=0 Pa  pressure_drop_nominal_specify=off  pressure_drop_nominal_unit=Pa  pressure_drop_nominal_value=1  flow_rate_specify=off  flow_rate_priority=None  flow_rate=0 m^3/s  flow_rate_nominal_specify=off  flow_rate_nominal_unit=m^3/s  flow_rate_nominal_value=1
      settings: SourceProductBaseCode=SH  InternalSimscapePortConfiguration="{\"Bottom\":[],\"Left\":[{\"id\":\"A\",\"label\":\"A\",\"type\":\"foundation.hydraulic.hydraulic\"}],\"Right\":[{\"id\":\"B\",\"label\":\"B\",\"type\":\"foundation.hydraulic.hydraulic\"}],\"Top\":[]}"
  Pump 1 : sh_lib/Pumps and Motors/Centrifugal Pump  mdl_type=2  c_1=326.8 Pa/(kg/m^3)  c_2=3.104e+04 Pa*s/kg  c_3=1.097e+07 Pa*s^2/(kg*m^3)  c_4=2.136e+05 Pa*s^2/(kg*m^3)  c_f=0.8  design_del=130 lpm  ref_velocity=1.77e+03 rpm  ref_density=1000 kg/m^3  leak_resistance=1e+8 Pa/(m^3/s)  T_const=0.1 N*m  trq_press_coeff=1e-6 N*m/Pa  pump_del_1D="[0    0.0032    0.0063    0.0095    0.0126    0.0158] m^3/s"  press_diff_1D="[4.4851    4.3655    4.1413    3.7376    2.9901    1.7940] bar"  pump_del_power_1D="[0    0.0032    0.0063    0.0095    0.0126    0.0158] m^3/s"  power_1D="[0\t2116.60000000000\t3727.20000000000\t4734.30000000000\t5232.70000000000\t4360.90000000000] W"  pump_vel_2D="[  3.2e+03 3.3e+03 3.4e+03 3.5e+03 ] rpm"  pump_del_2D="[  0 50 100 150 200 250 300 350 ] lpm"  press_diff_2D="[  8.3 8.8 9.3 9.9 ; 7.8 8.3 8.8 9.4 ; 7.2 7.6 8.2 8.7 ; 6.5 7 7.5 8 ; 5.6 6.1 6.6 7.1 ; 4.7 5.2 5.7 6.2 ; 3.4 4 4.4 4.9 ; 2.3 2.7 3.4 3.6 ; ] bar"  pump_del_power_2D="[  0 50 100 150 200 250 300 350 ] lpm"  power_2D="[  1.223e+03 1.341e+03 1.467e+03 1.6e+03 ; 1.414e+03 1.551e+03 1.696e+03 1.85e+03 ; 1.636e+03 1.794e+03 1.962e+03 2.14e+03 ; 1.941e+03 2.129e+03 2.326e+03 2.54e+03 ; 2.224e+03 2.439e+03 2.66e+03 2.91e+03 ; 2.453e+03 2.691e+03 2.947e+03 3.21e+03 ; 2.757e+03 3.024e+03 3.307e+03 3.608e+03 ; 2.945e+03 3.23e+03 3.533e+03 3.854e+03 ; ] W"  omega_threshold=1e-9 rad/s  interp_method=2  extrap_method=1
      settings: SourceProductBaseCode=SH  InternalSimscapePortConfiguration="{\"Bottom\":[],\"Left\":[{\"id\":\"S\",\"label\":\"S\",\"type\":\"foundation.mechanical.rotational.rotational\"}],\"Right\":[{\"id\":\"P\",\"label\":\"P\",\"type\":\"foundation.hydraulic.hydraulic\"},{\"id\":\"T\",\"label\":\"T\",\"type\":\"foundation.hydraulic.hydraulic\"}],\"Top\":[]}"
  Scope : Scope
  Simulink-PS Converter1 : nesl_utility/Simulink-PS Converter  PhysicalDomain=network_engine_domain  SubClassName=ps_input  LeftPortType=input  RightPortType=output  PseudoPeriodic=off  Frequencies=[]  NoiseDistribution=none  NoiseParameters=[]  Unit=rpm  AffineConversion=off  FilteringAndDerivatives=zero  SimscapeFilterOrder=1  InputFilterTimeConstant=.001  UdotUserProvided=0
  Velocity Source Pump 1 : fl_lib/Mechanical/Mechanical Sources/Ideal Angular Velocity Source
  induction machine : Subsystem
  inletT : PMIOPort  Side=Left
  outletT : PMIOPort  Port=2  Side=Right
  wires:
  f/1 -> Drive and Amplifier Dynamics/1
  induction machine/1(w) -> Simulink-PS Converter1/1
  Drive and Amplifier Dynamics/1 -> induction machine/1(f)
  PS-Simulink Converter2/1 -> Scope/1
  connections:
  Velocity Source Pump 1/LConn1 -- Pump 1/LConn1
  MRRef Pump 1/LConn1 -- Velocity Source Pump 1/RConn2
  inletT/RConn1 -- Pump 1/RConn2
  Pipe P/LConn1 -- Pump 1/RConn1
  Simulink-PS Converter1/RConn1 -- Velocity Source Pump 1/RConn1
  Pipe P/RConn1 -- Hydraulic Flow Rate Sensor/LConn1
  Hydraulic Flow Rate Sensor/RConn2 -- outletT/RConn1
  PS-Simulink Converter2/LConn1 -- Hydraulic Flow Rate Sensor/RConn1

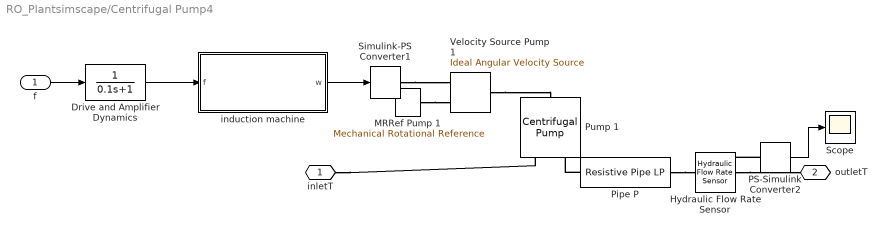
== system RO_Plantsimscape/Centrifugal Pump4 ==
  f : Inport
  Drive and Amplifier Dynamics : TransferFcn  Denominator=[0.1 1]
  Hydraulic Flow Rate Sensor : fl_lib/Hydraulic/Hydraulic Sensors/Hydraulic Flow Rate Sensor
  MRRef Pump 1 : fl_lib/Mechanical/Rotational Elements/Mechanical Rotational Reference
  PS-Simulink Converter2 : nesl_utility/PS-Simulink Converter  PhysicalDomain=network_engine_domain  SubClassName=ps_output  LeftPortType=input  RightPortType=output  PseudoPeriodic=off  Frequencies=[]  Unit=1  AffineConversion=off
  Pipe P : sh_lib/Low-Pressure Blocks/Resistive Pipe LP  cs_type=1  d_in=112.1660 mm  area=1e-04 m^2  D_h=0.0112 m  s_factor=64  length=8.1 m  length_ad=1 m  roughness=0.005 mm  Re_lam=2e+03  Re_turb=4e+03  elevation_A=45 m  elevation_B=45 m  g=9.80665 m/s^2  pressure_drop_specify=off  pressure_drop_priority=None  pressure_drop=0 Pa  pressure_drop_nominal_specify=off  pressure_drop_nominal_unit=Pa  pressure_drop_nominal_value=1  flow_rate_specify=off  flow_rate_priority=None  flow_rate=0 m^3/s  flow_rate_nominal_specify=off  flow_rate_nominal_unit=m^3/s  flow_rate_nominal_value=1
      settings: SourceProductBaseCode=SH  InternalSimscapePortConfiguration="{\"Bottom\":[],\"Left\":[{\"id\":\"A\",\"label\":\"A\",\"type\":\"foundation.hydraulic.hydraulic\"}],\"Right\":[{\"id\":\"B\",\"label\":\"B\",\"type\":\"foundation.hydraulic.hydraulic\"}],\"Top\":[]}"
  Pump 1 : sh_lib/Pumps and Motors/Centrifugal Pump  mdl_type=2  c_1=326.8 Pa/(kg/m^3)  c_2=3.104e+04 Pa*s/kg  c_3=1.097e+07 Pa*s^2/(kg*m^3)  c_4=2.136e+05 Pa*s^2/(kg*m^3)  c_f=0.8  design_del=130 lpm  ref_velocity=1.77e+03 rpm  ref_density=1000 kg/m^3  leak_resistance=1e+8 Pa/(m^3/s)  T_const=0.1 N*m  trq_press_coeff=1e-6 N*m/Pa  pump_del_1D="[0    0.0032    0.0063    0.0095    0.0126    0.0158] m^3/s"  press_diff_1D="[4.4851    4.3655    4.1413    3.7376    2.9901    1.7940] bar"  pump_del_power_1D="[0    0.0032    0.0063    0.0095    0.0126    0.0158] m^3/s"  power_1D="[0\t2116.60000000000\t3727.20000000000\t4734.30000000000\t5232.70000000000\t4360.90000000000] W"  pump_vel_2D="[  3.2e+03 3.3e+03 3.4e+03 3.5e+03 ] rpm"  pump_del_2D="[  0 50 100 150 200 250 300 350 ] lpm"  press_diff_2D="[  8.3 8.8 9.3 9.9 ; 7.8 8.3 8.8 9.4 ; 7.2 7.6 8.2 8.7 ; 6.5 7 7.5 8 ; 5.6 6.1 6.6 7.1 ; 4.7 5.2 5.7 6.2 ; 3.4 4 4.4 4.9 ; 2.3 2.7 3.4 3.6 ; ] bar"  pump_del_power_2D="[  0 50 100 150 200 250 300 350 ] lpm"  power_2D="[  1.223e+03 1.341e+03 1.467e+03 1.6e+03 ; 1.414e+03 1.551e+03 1.696e+03 1.85e+03 ; 1.636e+03 1.794e+03 1.962e+03 2.14e+03 ; 1.941e+03 2.129e+03 2.326e+03 2.54e+03 ; 2.224e+03 2.439e+03 2.66e+03 2.91e+03 ; 2.453e+03 2.691e+03 2.947e+03 3.21e+03 ; 2.757e+03 3.024e+03 3.307e+03 3.608e+03 ; 2.945e+03 3.23e+03 3.533e+03 3.854e+03 ; ] W"  omega_threshold=1e-9 rad/s  interp_method=2  extrap_method=1
      settings: SourceProductBaseCode=SH  InternalSimscapePortConfiguration="{\"Bottom\":[],\"Left\":[{\"id\":\"S\",\"label\":\"S\",\"type\":\"foundation.mechanical.rotational.rotational\"}],\"Right\":[{\"id\":\"P\",\"label\":\"P\",\"type\":\"foundation.hydraulic.hydraulic\"},{\"id\":\"T\",\"label\":\"T\",\"type\":\"foundation.hydraulic.hydraulic\"}],\"Top\":[]}"
  Scope : Scope
  Simulink-PS Converter1 : nesl_utility/Simulink-PS Converter  PhysicalDomain=network_engine_domain  SubClassName=ps_input  LeftPortType=input  RightPortType=output  PseudoPeriodic=off  Frequencies=[]  NoiseDistribution=none  NoiseParameters=[]  Unit=rpm  AffineConversion=off  FilteringAndDerivatives=zero  SimscapeFilterOrder=1  InputFilterTimeConstant=.001  UdotUserProvided=0
  Velocity Source Pump 1 : fl_lib/Mechanical/Mechanical Sources/Ideal Angular Velocity Source
  induction machine : Subsystem
  inletT : PMIOPort  Side=Left
  outletT : PMIOPort  Port=2  Side=Right
  wires:
  f/1 -> Drive and Amplifier Dynamics/1
  induction machine/1(w) -> Simulink-PS Converter1/1
  Drive and Amplifier Dynamics/1 -> induction machine/1(f)
  PS-Simulink Converter2/1 -> Scope/1
  connections:
  Velocity Source Pump 1/LConn1 -- Pump 1/LConn1
  MRRef Pump 1/LConn1 -- Velocity Source Pump 1/RConn2
  inletT/RConn1 -- Pump 1/RConn2
  Pipe P/LConn1 -- Pump 1/RConn1
  Simulink-PS Converter1/RConn1 -- Velocity Source Pump 1/RConn1
  Pipe P/RConn1 -- Hydraulic Flow Rate Sensor/LConn1
  Hydraulic Flow Rate Sensor/RConn2 -- outletT/RConn1
  PS-Simulink Converter2/LConn1 -- Hydraulic Flow Rate Sensor/RConn1
